simulink model "cstr_y"  (R2020b)
settings: Solver=ode15s  StartTime=0.0  StopTime=1200  RelTol=1e-8  EnableMultiTasking=on
libraries: simulink x6, pid_lib x1
settings Model: Creator=Karl  LastModifiedBy=Fuzz4
settings DataIOCC: SaveFormat=Array  ReturnWorkspaceOutputs=off  OutputOption=SpecifiedOutputTimes  OutputTimes=[0:1200]
settings OptimizationCC: LifeSpan=inf
settings DebuggingCC: UnderspecifiedInitializationDetection=Classic  MergeDetectMultiDrivingBlocksExec=none  SFUnexpectedBacktrackingDiag=warning  SFNoUnconditionalDefaultTransitionDiag=warning  SFExecutionAtInitializationDiag=none  ArithmeticOperatorsInVariantConditions=warning
settings HardwareCC: ProdBitPerPointer=32  ProdBitPerSizeT=32  ProdBitPerPtrDiffT=32  ProdLargestAtomicFloat=None  ProdIntDivRoundTo=Undefined  ProdEndianess=Unspecified  ProdWordSize=32  ProdHWDeviceType=32-bit Generic
settings ModelReferenceCC: PropagateSignalLabelsOutOfModel=off
settings SFSimCC: SimUseLocalCustomCode=off  CustomCodeUndefinedFunction=UseInterfaceOnly
settings RTWCC: RTWUseLocalCustomCode=off
settings CodeAppCC: StateflowObjectComments=on
settings GRTTargetCC: TargetLangStandard=C89/C90 (ANSI)
settings ConfigComp: CovMetricSettings=dw  CovSaveCumulativeToWorkspaceVar=on  CovSaveSingleToWorkspaceVar=on  CovExternalEMLEnable=off

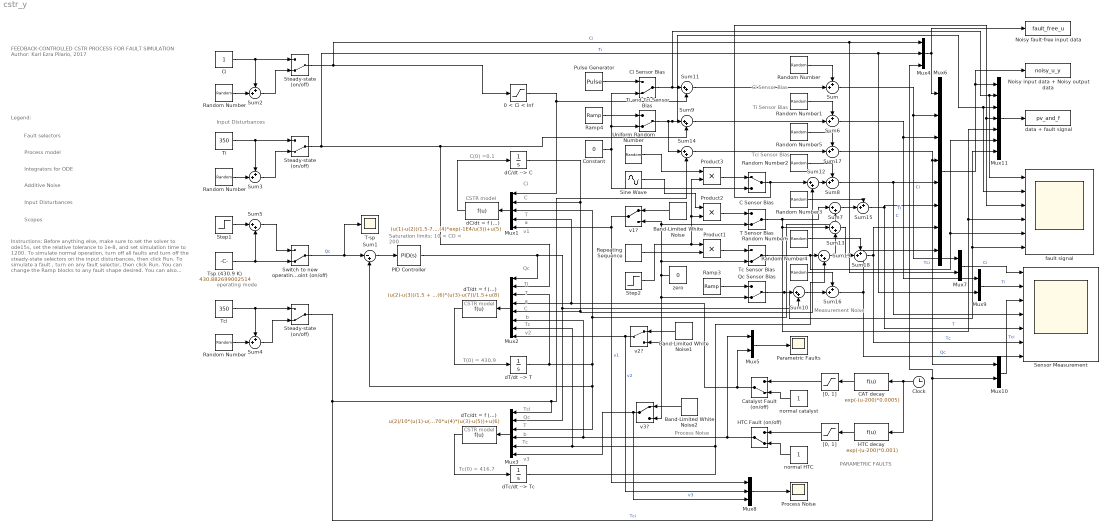
== system cstr_y ==
  note: Tci Sensor Bias
  note: Ti Sensor Bias
  note: Ci Sensor Bias
  note: Scopes
  note: Input Disturbances
  note: Instructions:
      |
      | Before anything else, make sure to set the solver to ode15s, set the relative tolerance to 1e-8, and set simulation time to 1200.
      |
      | To simulate normal operation, turn off all faults and turn off the steady-state selectors on the input disturbances, then click Run.
      |
      | To simulate a fault , turn on any fault selector, then click Run. You can change the Ramp blocks to any fault shape desired. You can also induce different disturbances by changing the Random Number blocks.
      |
      | Process Model:
  note: Additive Noise
  note: Integrators for ODE
  note: Process model
  note: Fault selectors
  note: Legend:
  note: FEEDBACK-CONTROLLED
      | CSTR PROCESS FOR
      | FAULT SIMULATION
      |
      | Author: Karl Ezra Pilario, 2017
  note: PARAMETRIC FAULTS
  note: v3
  note: v2
  note: v1
  note: T
  note: Tc(0) = 416.7
  note: Tc
  note: Qc
  note: Tc
  note: b
  note: Tci
  note: T
  note: Saturation limits:
      |  10 < CO < 200
  note: b
  note: CSTR model
  note: CSTR model
  note: T(0) = 430.9
  note: C(0) =0.1
  note: Measurement
      |         Noise
  note: Qc
  note: C
  note: a
  note: T
  note: Ti
  note: a
  note: C
  note: Ci
  note: CSTR model
  note: Process Noise
  note: Input Disturbances
  note: operating mode
  "   Steady-state (on/off)" : ManualSwitch  CurrentSetting=0
  "  Steady-state (on/off)" : ManualSwitch  CurrentSetting=0
  " Parametric Faults" : Scope
  " Process Noise" : Scope
  " Random Number" : RandomNumber  Variance=2  Seed=randi(100000)  SampleTime=60
  " [0, 1]" : Saturate  UpperLimit=1  LowerLimit=0
  0 < Ci < Inf : Saturate  UpperLimit=Inf  LowerLimit=0
  Band-Limited White Noise : simulink/Sources/Band-Limited White Noise  Cov=[1e-4]  Ts=1  seed=randi(100000)
  Band-Limited White Noise1 : simulink/Sources/Band-Limited White Noise  Cov=[1e-4]  Ts=1  seed=randi(100000)
  Band-Limited White Noise2 : simulink/Sources/Band-Limited White Noise  Cov=[1e-4]  Ts=1  seed=randi(100000)
  C Sensor Bias : ManualSwitch
  CAT decay : Fcn  Expr=exp(-(u-200)*0.0005)
  Catalyst Fault (on/off) : ManualSwitch  CurrentSetting=0
  Ci : Constant
  Ci Sensor Bias : ManualSwitch  CurrentSetting=0
  Clock : Clock
  Constant : Constant  Value=0
  HTC Fault (on/off) : ManualSwitch  CurrentSetting=0
  HTC decay : Fcn  Expr=exp(-(u-200)*0.001)
  Mux1 : Mux  Inputs=5
  Mux{5,7,9..10} (4 alike) : Mux  Inputs=2
  Mux11 : Mux  Inputs=7
  Mux2 : Mux  Inputs=8
  Mux3 : Mux  Inputs=6
  Mux4 : Mux  Inputs=3
  Mux6 : Mux  Inputs=8
  Mux8 : Mux  Inputs=3
  Noisy fault-free input data : ToWorkspace  VariableName=fault_free_u  SampleTime=1
  Noisy input data + Noisy output data : ToWorkspace  VariableName=noisy_u_y  SampleTime=-1
  PID Controller : pid_lib/PID Controller  Controller=PID  Form=Parallel  TimeDomain=Continuous-time  UseExternalTs=off  SampleTime=-1  IntegratorMethod=Forward Euler  FilterMethod=Forward Euler  ControllerParametersSource=internal  P=1  I=5  D=0  UseFilter=on  N=100  TunerSelectOption=Transfer Function Based (PID Tuner App)  InitialConditionSource=internal  InitialConditionForIntegrator=148.550238092053  InitialConditionForFilter=0  DifferentiatorICPrevScaledInput=0  ExternalReset=none  TrackingMode=off  Kt=1  LimitOutput=on  SatLimitsSource=internal  UpperSaturationLimit=200  LowerSaturationLimit=10  LinearizeAsGain=on  AntiWindupMode=none  Kb=1  POutMin=[]  POutMax=[]  IOutMin=[]  IOutMax=[]  DOutMin=[]  DOutMax=[]  NOutMin=[]  NOutMax=[]  SumOutMin=[]  SumOutMax=[]  SaturationOutMin=[]  SaturationOutMax=[]  PParamMin=[]  PParamMax=[]  IParamMin=[]  IParamMax=[]  DParamMin=[]  DParamMax=[]  NParamMin=[]  NParamMax=[]  KbParamMin=[]  KbParamMax=[]  KtParamMin=[]  KtParamMax=[]  KbOutMin=[]  KbOutMax=[]  KtOutMin=[]  KtOutMax=[]  IntegratorOutMin=[]  IntegratorOutMax=[]  FilterOutMin=[]  FilterOutMax=[]  SumI1OutMin=[]  SumI1OutMax=[]  SumI2OutMin=[]  SumI2OutMax=[]  SumI3OutMin=[]  SumI3OutMax=[]  SumI4OutMin=[]  SumI4OutMax=[]  SumDOutMin=[]  SumDOutMax=[]  DifferentiatorOutMin=[]  DifferentiatorOutMax=[]  FilterDiffOutCoefMin=[]  FilterDiffOutCoefMax=[]  ReciprocalOutMin=[]  ReciprocalOutMax=[]  SumDenOutMin=[]  SumDenOutMax=[]  SumNumOutMin=[]  SumNumOutMax=[]  DivideOutMin=[]  DivideOutMax=[]  UdiffTsProdOutMin=[]  UdiffTsProdOutMax=[]  NTsProdOutMin=[]  NTsProdOutMax=[]  UintegralTsProdOutMin=[]  UintegralTsProdOutMax=[]  UngainTsProdOutMin=[]  UngainTsProdOutMax=[]  IntegratorContinuousStateAttributes=''  IntegratorStateMustResolveToSignalObject=off  IntegratorRTWStateStorageClass=Auto  FilterContinuousStateAttributes=''  FilterStateMustResolveToSignalObject=off  FilterRTWStateStorageClass=Auto  ParallelPVariant=InternalParameters  IdealPVariant=Disabled  IVariant=InternalParameters  DVariant=InternalParameters  IntegratorVariant=Continuous  SatVariant=Enabled  AWVariant=Passthrough  PCopyVariant=Disabled  TRVariant=Disabled  FdbkBlocksVariant=Forward  IdealPFdbkVariant=Disabled  SatFdbkVariant=Disabled  DerivativeFilterVariant=ContFilter  NVariant=InternalParameters  NCopyVariant=Disabled  FilterICVariant=InternalICsFilter  IntegratorICVariant=InternalICs  ExternalResetVariant=Disabled  TRSumVariant=Passthrough  SumFdbkVariant=Disabled  SumVariant=Sum_PID  TsampFilterVariant=InternalTs  TsampNgainVariant=Passthrough  TsampIntegralVariant=Passthrough  ExternalSaturationOutDataTypeStr=Inherit: Same as second input
  Product1 : Product
  Product2 : Product
  Product3 : Product
  Pulse Generator : DiscretePulseGenerator  PulseType=Time based  Period=100  PulseWidth=50  PhaseDelay=200
  Qc Sensor Bias : ManualSwitch  CurrentSetting=0
  Ramp3 : simulink/Sources/Ramp  slope=-100/(1200-200)  start=200  InitialOutput=0
  Ramp4 : simulink/Sources/Ramp  slope=50/(1200-200)  start=200  InitialOutput=0
  Random Number : RandomNumber  Variance=0.000001  Seed=randi(100000)  SampleTime=1
  Random Number1 : RandomNumber  Variance=0.05  Seed=randi(100000)  SampleTime=1
  Random Number2 : RandomNumber  Variance=0.000001  Seed=randi(100000)  SampleTime=1
  Random Number3 : RandomNumber  Variance=0.001  Seed=randi(100000)  SampleTime=1
  Random Number4 : RandomNumber  Variance=0.2  Seed=randi(100000)  SampleTime=1
  Random Number5 : RandomNumber  Variance=0.05  Seed=randi(100000)  SampleTime=1
  Random Number6 : RandomNumber  Variance=0.05  Seed=randi(100000)  SampleTime=1
  Random Number : RandomNumber  Variance=2  Seed=randi(100000)  SampleTime=60
  Random Number : RandomNumber  Variance=0.002  Seed=randi(100000)  SampleTime=60
  Repeating Sequence : simulink/Sources/Repeating Sequence  rep_seq_t=[0 200]  rep_seq_y=[0 50]
  "Sensor Measurement " : Scope  NumInputPorts=7
  Sine Wave : Sin  Amplitude=50  Frequency=2*3.14159265/200  SampleTime=0
  Steady-state (on/off) : ManualSwitch  CurrentSetting=0
  Step1 : Step  Time=300  After=10  SampleTime=0
  Step2 : Step  Time=200  SampleTime=0
  Sum{,2..4,6,8,15..18} (10 alike) : Sum  Inputs=++|
  Sum1 : Sum  Inputs=|-+
  Sum{5,7,9..14,19} (9 alike) : Sum  Inputs=|++
  Switch to new operating point (on/off) : ManualSwitch  CurrentSetting=0
  T Sensor Bias : ManualSwitch  CurrentSetting=0
  T-sp : Scope
  Tc Sensor Bias : ManualSwitch  CurrentSetting=0
  Tci : Constant  Value=350
  Ti : Constant  Value=350
  Ti and Tci Sensor Bias : ManualSwitch  CurrentSetting=0
  Tsp (430.9 K) : Constant  Value=430.882699002514
  Uniform Random Number : UniformRandomNumber  SampleTime=1
  "[0, 1]" : Saturate  UpperLimit=1  LowerLimit=0
  dC/dt --> C : Integrator  InitialCondition=0.1
  dC/dt = f (...) : Fcn  Expr=(u(1)-u(2))/1.5-7.2E10*u(2)*u(4)*exp(-1E4/u(3))+u(5)
  dT/dt --> T : Integrator  InitialCondition=430.882699002514
  dT/dt = f (...) : Fcn  Expr=(u(2)-u(3))/1.5 + u(4)*7.2E10*exp(-1E4/u(3))*u(5)*2E2 - 7*u(6)*(u(3)-u(7))/1.5+u(8)
  dTc/dt --> Tc : Integrator  InitialCondition=416.723084574301
  dTc/dt = f (...) : Fcn  Expr=u(2)/10*(u(1)-u(5)) + 70*u(4)*(u(3)-u(5))+u(6)
  data + fault signal : ToWorkspace  VariableName=pv_and_f  SampleTime=-1
  fault signal : Scope  NumInputPorts=6
  normal catalyst : Constant
  normal HTC : Constant
  v1? : ManualSwitch
  v2? : ManualSwitch
  v3? : ManualSwitch
  zero : Constant  Value=0
  wires:
  dT/dt = f (...)/1 -> dT/dt --> T/1
  Mux1/1 -> dC/dt = f (...)/1
  Catalyst Fault (on/off)/1 -> Mux5/2, Mux1/4, Mux2/4
  Mux2/1 -> dT/dt = f (...)/1
  dT/dt --> T/1 -> Mux2/3, Mux1/3, Sum7/2, Mux3/3, Sum1/2
  Sum1/1 -> PID Controller/1
  CAT decay/1 -> "[0, 1]"/1
  Ci/1 -> Steady-state (on/off)/1, Sum2/1
  Ti/1 -> "  Steady-state (on/off)"/1, Sum3/1
  normal catalyst/1 -> Catalyst Fault (on/off)/2
  HTC Fault (on/off)/1 -> Mux5/1, Mux2/6, Mux3/4
  Sum2/1 -> Steady-state (on/off)/2
  Sum3/1 -> "  Steady-state (on/off)"/2
  Switch to new operating point (on/off)/1 -> T-sp/1, Sum1/1  "Qc"
  Tsp (430.9 K)/1 -> Sum5/2, Switch to new operating point (on/off)/2
  Clock/1 -> HTC decay/1, CAT decay/1
  HTC decay/1 -> " [0, 1]"/1
  Tci/1 -> "   Steady-state (on/off)"/1, Sum4/1
  Sum4/1 -> "   Steady-state (on/off)"/2
  Mux3/1 -> dTc/dt = f (...)/1
  dTc/dt = f (...)/1 -> dTc/dt --> Tc/1
  dTc/dt --> Tc/1 -> Sum19/2, Mux2/7, Mux3/5
  Sum18/1 -> "Sensor Measurement "/6, Mux6/7  "Tc"
  Sum17/1 -> Mux6/4, Mux10/1  "Tci"
  Sum16/1 -> Mux6/8, "Sensor Measurement "/7  "Qc"
  Mux6/1 -> Noisy input data + Noisy output data/1, Mux11/1
  Mux5/1 -> " Parametric Faults"/1
  Steady-state (on/off)/1 -> Mux4/1, Mux7/2, 0 < Ci < Inf/1  "Ci"
  Sum/1 -> Mux6/2, Mux7/1  "Ci"
  dC/dt --> C/1 -> Sum12/2, Mux2/5, Mux1/2
  Ramp4/1 -> Ti and Tci Sensor Bias/1
  dC/dt = f (...)/1 -> dC/dt --> C/1
  Ramp3/1 -> Qc Sensor Bias/1
  Sum11/1 -> Sum/2
  0 < Ci < Inf/1 -> Sum11/2, Mux1/1
  Sine Wave/1 -> Product2/1
  C Sensor Bias/1 -> Mux11/4, fault signal/3, Sum12/1
  Repeating Sequence/1 -> Product1/2
  Sum13/1 -> Sum18/2
  Sum5/1 -> Switch to new operating point (on/off)/1
  Step1/1 -> Sum5/1
  Mux8/1 -> " Process Noise"/1
  Band-Limited White Noise/1 -> v1?/1
  v1?/1 -> Mux8/1, Mux1/5  "v1"
  Band-Limited White Noise1/1 -> v2?/1
  v2?/1 -> Mux8/2, Mux2/8  "v2"
  Band-Limited White Noise2/1 -> v3?/1
  v3?/1 -> Mux8/3, Mux3/6  "v3"
  zero/1 -> Tc Sensor Bias/2, T Sensor Bias/2, v1?/2, Qc Sensor Bias/2, v3?/2, v2?/2
  normal HTC/1 -> HTC Fault (on/off)/2
  PID Controller/1 -> Sum10/2, Mux3/2, Mux2/1
  Random Number/1 -> Sum2/2
  Random Number/1 -> Sum3/2
  " Random Number"/1 -> Sum4/2
  " [0, 1]"/1 -> HTC Fault (on/off)/1
  "[0, 1]"/1 -> Catalyst Fault (on/off)/1
  Sum8/1 -> Mux6/5, "Sensor Measurement "/4  "C"
  Sum15/1 -> Mux6/6, "Sensor Measurement "/5  "T"
  Random Number/1 -> Sum/1
  Random Number1/1 -> Sum6/1
  Sum9/1 -> Sum6/2
  Sum6/1 -> Mux6/3, Mux9/1  "Ti"
  Random Number2/1 -> Sum8/1
  Sum7/1 -> Sum15/2
  Random Number3/1 -> Sum15/1
  Sum10/1 -> Sum16/2
  Random Number4/1 -> Sum16/1
  Sum14/1 -> Sum17/2
  Random Number5/1 -> Sum17/1
  Random Number6/1 -> Sum18/1
  "  Steady-state (on/off)"/1 -> Sum9/2, Mux2/2, Mux9/2, Mux4/2  "Ti"
  "   Steady-state (on/off)"/1 -> Mux3/1, Sum14/2, Mux4/3, Mux10/2  "Tci"
  Mux7/1 -> "Sensor Measurement "/1  "Ci"
  Mux9/1 -> "Sensor Measurement "/2  "Ti"
  Mux10/1 -> "Sensor Measurement "/3  "Tci"
  Mux4/1 -> Mux6/1, Noisy fault-free input data/1
  Constant/1 -> Ti and Tci Sensor Bias/2, Ci Sensor Bias/2, C Sensor Bias/2
  Ti and Tci Sensor Bias/1 -> Mux11/3, fault signal/2, Sum9/1, Sum14/1
  Ci Sensor Bias/1 -> fault signal/1, Mux11/2, Sum11/1
  T Sensor Bias/1 -> Sum13/1, Mux11/5, fault signal/4, Sum7/1
  Tc Sensor Bias/1 -> Mux11/6, fault signal/5, Sum19/1
  Sum19/1 -> Sum13/2
  Product1/1 -> Tc Sensor Bias/1
  Step2/1 -> Product2/2, Product3/2, Product1/1
  Pulse Generator/1 -> Ci Sensor Bias/1
  Sum12/1 -> Sum8/2
  Uniform Random Number/1 -> Product3/1
  Qc Sensor Bias/1 -> Mux11/7, fault signal/6, Sum10/1
  Mux11/1 -> data + fault signal/1
  Product2/1 -> T Sensor Bias/1
  Product3/1 -> C Sensor Bias/1
